simulink model "AutonomousCleaningSystemFunctionalArchitecture"  (R2022b)
settings: Solver=VariableStepAuto  StartTime=0.0  StopTime=10.0  RelTol=1e-3
settings Model: Creator=carol  LastModifiedBy=carol
settings OptimizationCC: ReuseModelBlockBuffer=on

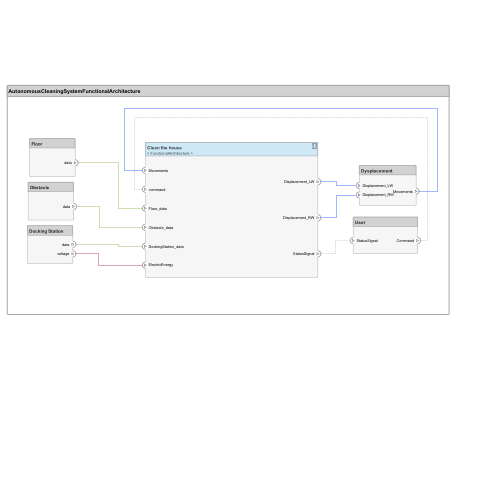
[thumbnail: Simulink's stored preview of the top-level diagram]
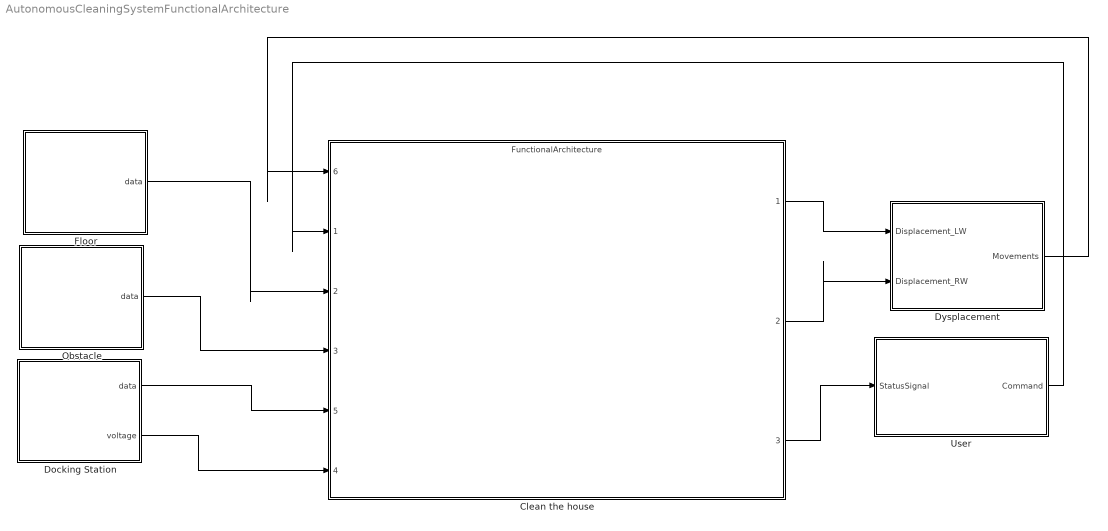
== system AutonomousCleaningSystemFunctionalArchitecture ==
  Clean the house : ModelReference  ModelNameDialog=FunctionalArchitecture  SimulationMode=Normal  ModelReferenceVersion=1.20
      settings: PortSchema="{\"entries\":[{\"content\":{\"headerSize\":38,\"margin\":15,\"minimumSpacing\":25,\"sides\":[{\"content\":{\"connectorIds\":[\"In6\",\"In1\",\"In2\",\"In3\",\"In5\",\"In4\"]},\"type\":\"ConnectorPlacement.EquallySpacedRectSide\",\"uuid\":\"49d8acf2-1330-494b-b046-2398c791023a\"},{\"content\":{\"connectorIds\":[\"Out1\",\"Out2\",\"Out3\"],\"side\":\"RIGHT\"},\"type\":\"ConnectorPlacement.EquallySpacedRectSide\",\"uuid\":\"c108b3f3-ffbe-42c6-96a6-f7277ca144e3\"},{\"content\":{\"side\":\"TOP\"},\"type\":\"ConnectorPlacement.EquallySpacedRectSide\",\"uuid\":\"8ab1d4b7-bc94-48f4-88b9-5774a0ab0845\"}]},\"type\":\"ConnectorPlacement.EquallySpacedConnector\",\"uuid\":\"2ac5de44-339a-4824-ba6a-4df3d648c111\"}],\"packageUris\":[\"http://schema.mathworks.com/mf0/Connector/R2020b\"],\"version\":\"1.0\"}"
  Docking Station : Subsystem
      settings: PortSchema="{\"entries\":[{\"content\":{\"headerSize\":26,\"margin\":15,\"minimumSpacing\":25,\"sides\":[{\"content\":{},\"type\":\"ConnectorPlacement.EquallySpacedRectSide\",\"uuid\":\"4363930a-608c-49b3-a552-25912bab4631\"},{\"content\":{\"connectorIds\":[\"Out1\",\"Out2\"],\"side\":\"RIGHT\"},\"type\":\"ConnectorPlacement.EquallySpacedRectSide\",\"uuid\":\"46b32956-08e1-442a-91b2-d83b199630ea\"},{\"content\":{\"side\":\"TOP\"},\"type\":\"ConnectorPlacement.EquallySpacedRectSide\",\"uuid\":\"ba364085-3ac2-4596-8832-357eb5446ff0\"}]},\"type\":\"ConnectorPlacement.EquallySpacedConnector\",\"uuid\":\"92fd45a1-4b9d-46f0-9585-9d2548d6ba77\"}],\"packageUris\":[\"http://schema.mathworks.com/mf0/Connector/R2020b\"],\"version\":\"1.0\"}"
  Dysplacement : Subsystem
      settings: PortSchema="{\"entries\":[{\"content\":{\"headerSize\":26,\"margin\":15,\"minimumSpacing\":25,\"sides\":[{\"content\":{\"connectorIds\":[\"In1\",\"In2\"]},\"type\":\"ConnectorPlacement.EquallySpacedRectSide\",\"uuid\":\"6ae6270c-bff4-4a0d-8fba-8fdec87b0a05\"},{\"content\":{\"connectorIds\":[\"Out1\"],\"side\":\"RIGHT\"},\"type\":\"ConnectorPlacement.EquallySpacedRectSide\",\"uuid\":\"f3a0045b-bb3b-40f9-afd5-e1537ff3eeca\"},{\"content\":{\"side\":\"TOP\"},\"type\":\"ConnectorPlacement.EquallySpacedRectSide\",\"uuid\":\"e89a58f2-90b0-468c-bb6a-95617af68e24\"}]},\"type\":\"ConnectorPlacement.EquallySpacedConnector\",\"uuid\":\"066eb43c-7b96-4660-9f29-628dd77a5b3b\"}],\"packageUris\":[\"http://schema.mathworks.com/mf0/Connector/R2020b\"],\"version\":\"1.0\"}"
  Floor : Subsystem
      settings: PortSchema="{\"entries\":[{\"content\":{\"headerSize\":26,\"margin\":15,\"minimumSpacing\":25,\"sides\":[{\"content\":{},\"type\":\"ConnectorPlacement.EquallySpacedRectSide\",\"uuid\":\"4363930a-608c-49b3-a552-25912bab4631\"},{\"content\":{\"connectorIds\":[\"Out1\"],\"side\":\"RIGHT\"},\"type\":\"ConnectorPlacement.EquallySpacedRectSide\",\"uuid\":\"46b32956-08e1-442a-91b2-d83b199630ea\"},{\"content\":{\"side\":\"TOP\"},\"type\":\"ConnectorPlacement.EquallySpacedRectSide\",\"uuid\":\"ba364085-3ac2-4596-8832-357eb5446ff0\"}]},\"type\":\"ConnectorPlacement.EquallySpacedConnector\",\"uuid\":\"92fd45a1-4b9d-46f0-9585-9d2548d6ba77\"}],\"packageUris\":[\"http://schema.mathworks.com/mf0/Connector/R2020b\"],\"version\":\"1.0\"}"
  Obstacle : Subsystem
      settings: PortSchema="{\"entries\":[{\"content\":{\"headerSize\":26,\"margin\":15,\"minimumSpacing\":25,\"sides\":[{\"content\":{},\"type\":\"ConnectorPlacement.EquallySpacedRectSide\",\"uuid\":\"4363930a-608c-49b3-a552-25912bab4631\"},{\"content\":{\"connectorIds\":[\"Out1\"],\"side\":\"RIGHT\"},\"type\":\"ConnectorPlacement.EquallySpacedRectSide\",\"uuid\":\"46b32956-08e1-442a-91b2-d83b199630ea\"},{\"content\":{\"side\":\"TOP\"},\"type\":\"ConnectorPlacement.EquallySpacedRectSide\",\"uuid\":\"ba364085-3ac2-4596-8832-357eb5446ff0\"}]},\"type\":\"ConnectorPlacement.EquallySpacedConnector\",\"uuid\":\"92fd45a1-4b9d-46f0-9585-9d2548d6ba77\"}],\"packageUris\":[\"http://schema.mathworks.com/mf0/Connector/R2020b\"],\"version\":\"1.0\"}"
  User : Subsystem
      settings: PortSchema="{\"entries\":[{\"content\":{\"headerSize\":26,\"margin\":15,\"minimumSpacing\":25,\"sides\":[{\"content\":{\"connectorIds\":[\"In1\"]},\"type\":\"ConnectorPlacement.EquallySpacedRectSide\",\"uuid\":\"4363930a-608c-49b3-a552-25912bab4631\"},{\"content\":{\"connectorIds\":[\"Out1\"],\"side\":\"RIGHT\"},\"type\":\"ConnectorPlacement.EquallySpacedRectSide\",\"uuid\":\"46b32956-08e1-442a-91b2-d83b199630ea\"},{\"content\":{\"side\":\"TOP\"},\"type\":\"ConnectorPlacement.EquallySpacedRectSide\",\"uuid\":\"ba364085-3ac2-4596-8832-357eb5446ff0\"}]},\"type\":\"ConnectorPlacement.EquallySpacedConnector\",\"uuid\":\"92fd45a1-4b9d-46f0-9585-9d2548d6ba77\"}],\"packageUris\":[\"http://schema.mathworks.com/mf0/Connector/R2020b\"],\"version\":\"1.0\"}"
  wires:
  User/1(Command) -> Clean the house/1
  Floor/1(data) -> Clean the house/2
  Obstacle/1(data) -> Clean the house/3
  Docking Station/2(voltage) -> Clean the house/4
  Docking Station/1(data) -> Clean the house/5
  Clean the house/1 -> Dysplacement/1(Displacement_LW)
  Clean the house/2 -> Dysplacement/2(Displacement_RW)
  Dysplacement/1(Movements) -> Clean the house/6
  Clean the house/3 -> User/1(StatusSignal)

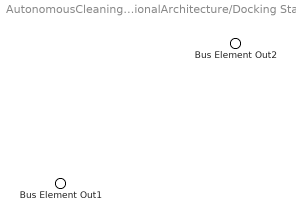
== system AutonomousCleaningSystemFunctionalArchitecture/Docking Station ==
  Bus Element Out2 : Outport  PortName=data
  Bus Element Out1 : Outport  Port=2  PortName=voltage

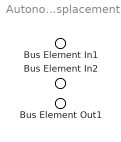
== system AutonomousCleaningSystemFunctionalArchitecture/Dysplacement ==
  Bus Element In1 : Inport  PortName=Displacement_LW
  Bus Element In2 : Inport  Port=2  PortName=Displacement_RW
  Bus Element Out1 : Outport  PortName=Movements

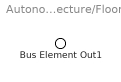
== system AutonomousCleaningSystemFunctionalArchitecture/Floor ==
  Bus Element Out1 : Outport  PortName=data

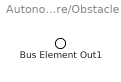
== system AutonomousCleaningSystemFunctionalArchitecture/Obstacle ==
  Bus Element Out1 : Outport  PortName=data

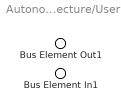
== system AutonomousCleaningSystemFunctionalArchitecture/User ==
  Bus Element In1 : Inport  PortName=StatusSignal
  Bus Element Out1 : Outport  PortName=Command
